simulink model "AppMainTest"  (R2019a)
settings: Solver=FixedStepDiscrete  StartTime=0.0  StopTime=300  FixedStep=1e-3  RelTol=1e-3
libraries: simulink x5
settings Model: Creator=mdl4347  LastModifiedBy=mdl4347
settings DebuggingCC: ModelReferenceIOMsg=warning

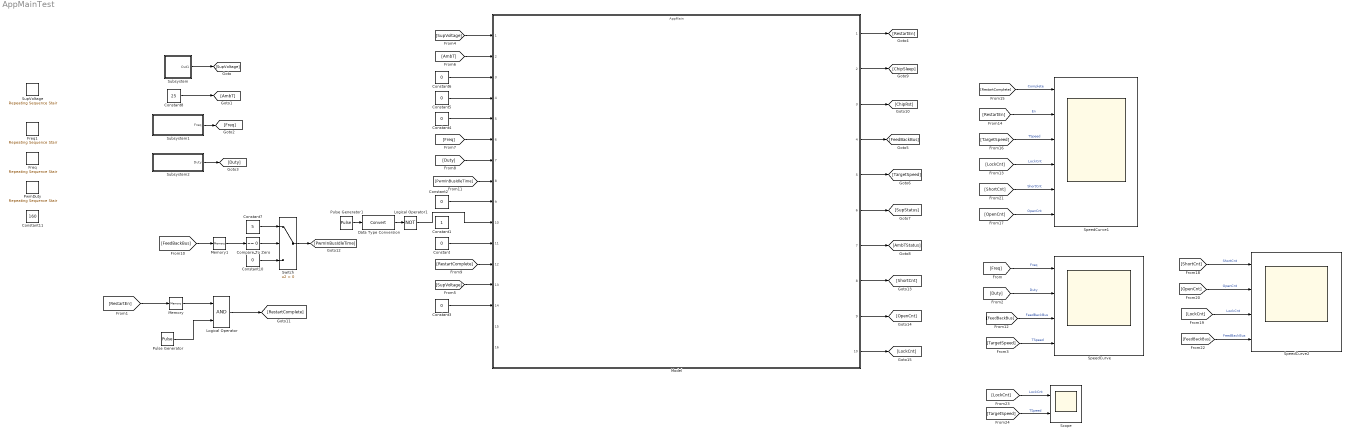
== system AppMainTest ==
  Compare To Zero : simulink/Logic and Bit Operations/Compare To Zero  relop===  OutDataTypeStr=boolean
  Constant{,2..6} (6 alike) : Constant  Value=0  OutDataTypeStr=boolean
  Constant1 : Constant  OutDataTypeStr=boolean
  Constant10 : Constant  Value=0  OutDataTypeStr=uint16
  Constant11 : Constant  Value=160
  Constant7 : Constant  Value=5  OutDataTypeStr=uint16
  Constant8 : Constant  Value=25  OutDataTypeStr=int16
  Data Type Conversion : DataTypeConversion
  Freq : simulink/Sources/Repeating Sequence Stair  OutValues=[480:1:520 520:-1:480 4980:1:5020 5020:-1:4980 4980:-10:480]  tsamp=50e-3  OutMin=[]  OutMax=[]  OutDataTypeStr=double  OutputDataTypeScalingMode=double  OutDataType=fixdt(0,8)  ConRadixGroup=Best Precision: Vector-wise  OutScaling=2^-12
  Freq1 : simulink/Sources/Repeating Sequence Stair  OutValues=[2000 6000]  tsamp=2  OutMin=[]  OutMax=[]  OutDataTypeStr=double  OutputDataTypeScalingMode=double  OutDataType=fixdt(0,8)  ConRadixGroup=Best Precision: Vector-wise  OutScaling=2^-12
  Logical Operator : Logic  AllPortsSameDT=off  OutDataTypeStr=boolean
  Logical Operator1 : Logic  Operator=NOT  AllPortsSameDT=off  OutDataTypeStr=boolean
  Memory : Memory  InheritSampleTime=on
  Memory1 : Memory  InitialCondition=1
  Model : ModelReference  ModelNameDialog=AppMain.slx  SimulationMode=Normal  ModelReferenceVersion=1.1070
  Pulse Generator : DiscretePulseGenerator  PulseType=Time based  Period=5  PulseWidth=0.1
  Pulse Generator1 : DiscretePulseGenerator  PulseType=Time based  Period=150  PulseWidth=3
  PwmDuty : simulink/Sources/Repeating Sequence Stair  OutValues=[0:10:1000 1000:-10:0]  tsamp=50e-3  OutMin=[]  OutMax=[]  OutDataTypeStr=double  OutputDataTypeScalingMode=double  OutDataType=fixdt(0,8)  ConRadixGroup=Best Precision: Vector-wise  OutScaling=2^-12
  Scope : Scope  NumInputPorts=2
  SpeedCurve : Scope  NumInputPorts=4
  SpeedCurve1 : Scope  NumInputPorts=6
  SpeedCurve2 : Scope  NumInputPorts=4
  Subsystem : Subsystem
  Subsystem1 : Subsystem
  Subsystem2 : Subsystem
  SupVoltage : simulink/Sources/Repeating Sequence Stair  OutValues=[240 160 159 170 171 320 321 310 309 ]  tsamp=1.5  OutMin=[]  OutMax=[]  OutDataTypeStr=double  OutputDataTypeScalingMode=double  OutDataType=fixdt(0,8)  ConRadixGroup=Best Precision: Vector-wise  OutScaling=2^-12
  Switch : Switch  Criteria=u2 > Threshold
  wires:
  Constant/1 -> Model/11
  Data Type Conversion/1 -> Logical Operator1/1
  Constant2/1 -> Model/9
  Constant4/1 -> Model/5
  Constant5/1 -> Model/4
  Constant6/1 -> Model/3
  Constant8/1 -> [AmbT]
  [PwmInBusIdleTime] -> Model/8
  Constant3/1 -> Model/14
  Model/1 -> [RestartEn]
  Model/4 -> [FeedBackBus]
  Model/5 -> [TargetSpeed]
  Model/6 -> [SupStatus]
  Model/7 -> [AmbTStatus]
  [RestartEn] -> Memory/1
  [Freq] -> SpeedCurve/1  "Freq"
  [Duty] -> SpeedCurve/2  "Duty"
  [TargetSpeed] -> SpeedCurve/4  "TSpeed"
  Model/2 -> [ChipSleep]
  Model/3 -> [ChipRst]
  [SupVoltage] -> Model/1
  [SupVoltage] -> Model/13
  [AmbT] -> Model/2
  [Freq] -> Model/6
  [Duty] -> Model/7
  [RestartComplete] -> Model/12
  Subsystem/1(Out1) -> [SupVoltage]
  Subsystem1/1(Freq) -> [Freq]
  Subsystem2/1(Duty) -> [Duty]
  [FeedBackBus] -> Memory1/1
  Memory1/1 -> Compare To Zero/1
  Compare To Zero/1 -> Switch/2
  Constant7/1 -> Switch/1
  Constant10/1 -> Switch/3
  Switch/1 -> [PwmInBusIdleTime]
  [FeedBackBus] -> SpeedCurve/3  "FeedBackBus"
  [TargetSpeed] -> SpeedCurve1/3  "TSpeed"
  [RestartEn] -> SpeedCurve1/2  "En"
  [RestartComplete] -> SpeedCurve1/1  "Complete"
  Model/8 -> [ShortCnt]
  Model/9 -> [OpenCnt]
  Model/10 -> [LockCnt]
  Pulse Generator/1 -> Logical Operator/2
  Logical Operator/1 -> [RestartComplete]
  Memory/1 -> Logical Operator/1
  [LockCnt] -> SpeedCurve1/4  "LockCnt"
  [OpenCnt] -> SpeedCurve1/6  "OpenCnt"
  [ShortCnt] -> SpeedCurve1/5  "ShortCnt"
  [LockCnt] -> SpeedCurve2/3  "LockCnt"
  [OpenCnt] -> SpeedCurve2/2  "OpenCnt"
  [ShortCnt] -> SpeedCurve2/1  "ShortCnt"
  [FeedBackBus] -> SpeedCurve2/4  "FeedBackBus"
  Pulse Generator1/1 -> Data Type Conversion/1
  Logical Operator1/1 -> Model/10
  [LockCnt] -> Scope/1  "LockCnt"
  [TargetSpeed] -> Scope/2  "TSpeed"

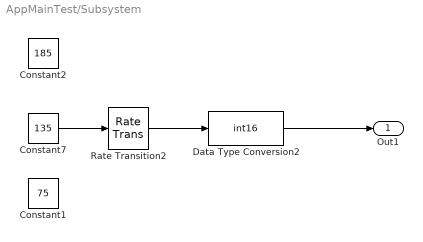
== system AppMainTest/Subsystem ==
  Constant1 : Constant  Value=75
  Constant2 : Constant  Value=185
  Constant7 : Constant  Value=135
  Data Type Conversion2 : DataTypeConversion  OutDataTypeStr=int16
  Rate Transition2 : RateTransition  OutPortSampleTime=10e-3
  Out1 : Outport
  wires:
  Rate Transition2/1 -> Data Type Conversion2/1
  Constant7/1 -> Rate Transition2/1
  Data Type Conversion2/1 -> Out1/1

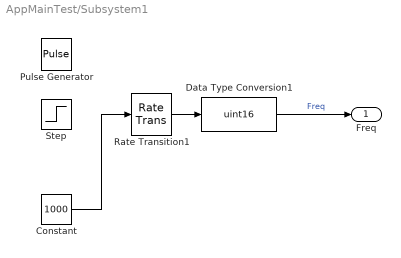
== system AppMainTest/Subsystem1 ==
  Constant : Constant  Value=1000
  Data Type Conversion1 : DataTypeConversion  OutDataTypeStr=uint16
  Pulse Generator : DiscretePulseGenerator  PulseType=Time based  Amplitude=1000  Period=5  PulseWidth=50
  Rate Transition1 : RateTransition  OutPortSampleTime=5e-3
  Step : Step  Time=5  Before=1000  After=1000  SampleTime=0
  Freq : Outport
  wires:
  Rate Transition1/1 -> Data Type Conversion1/1
  Constant/1 -> Rate Transition1/1
  Data Type Conversion1/1 -> Freq/1  "Freq"

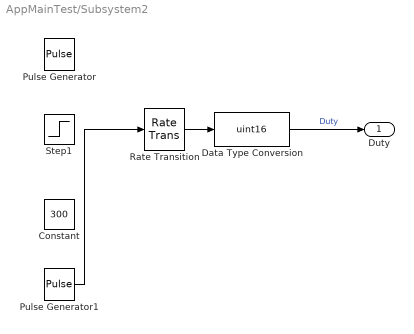
== system AppMainTest/Subsystem2 ==
  Constant : Constant  Value=300
  Data Type Conversion : DataTypeConversion  OutDataTypeStr=uint16
  Pulse Generator : DiscretePulseGenerator  PulseType=Time based  Amplitude=300  Period=5  PulseWidth=60%
  Pulse Generator1 : DiscretePulseGenerator  PulseType=Time based  Amplitude=300  Period=100  PulseWidth=90%
  Rate Transition : RateTransition  OutPortSampleTime=5e-3
  Step1 : Step  Time=6  Before=100  After=200  SampleTime=0
  Duty : Outport
  wires:
  Rate Transition/1 -> Data Type Conversion/1
  Pulse Generator1/1 -> Rate Transition/1
  Data Type Conversion/1 -> Duty/1  "Duty"
